simulink model "ex5"  (R2015a)
settings: Solver=ode45  StartTime=0.0  StopTime=100  RelTol=1e-3
values from neighbouring files (symbols this model uses):
  Kx = Kmpc(1,[1 2])    [ex5.m]
  Ky = Kmpc(1,3)    [ex5.m]
  r = 1    [ex5.m]
undefined symbols (not defined in the file or in its folder): Ad, Bd, Cd
libraries: simulink x1
settings Model: Creator=Xrisostomos  LastModifiedBy=Xrisostomos

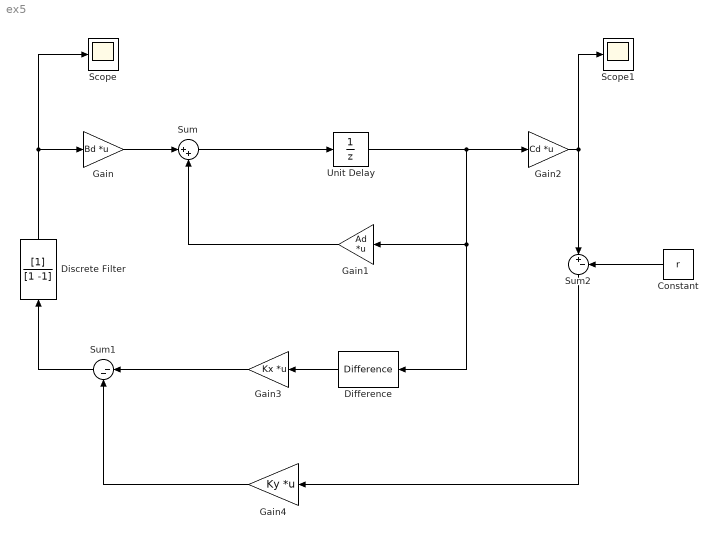
== system ex5 ==
  Constant : Constant  Value=r
  Difference : simulink/Discrete/Difference  ICPrevInput=0.0  InputProcessing=Inherited  OutMin=[]  OutMax=[]  OutDataType=fixdt(1, 16)  OutScaling=2^-10  DoSatur=off
  Discrete Filter : DiscreteFilter  Denominator=[1 -1]  SampleTime=2
  Gain : Gain  Gain=Bd  Multiplication=Matrix(K*u)
  Gain1 : Gain  Gain=Ad  Multiplication=Matrix(K*u)
  Gain2 : Gain  Gain=Cd  Multiplication=Matrix(K*u)
  Gain3 : Gain  Gain=Kx  Multiplication=Matrix(K*u)
  Gain4 : Gain  Gain=Ky  Multiplication=Matrix(K*u)
  Scope : Scope
  Scope1 : Scope
  Sum : Sum  Inputs=|++
  Sum1 : Sum  Inputs=|--
  Sum2 : Sum  Inputs=|+-
  Unit Delay : UnitDelay  SampleTime=-1
  wires:
  Gain1/1 -> Sum/2
  Sum/1 -> Unit Delay/1
  Unit Delay/1 -> Gain2/1, Difference/1, Gain1/1
  Difference/1 -> Gain3/1
  Gain3/1 -> Sum1/1
  Sum1/1 -> Discrete Filter/1
  Discrete Filter/1 -> Scope/1, Gain/1
  Gain/1 -> Sum/1
  Gain4/1 -> Sum1/2
  Constant/1 -> Sum2/2
  Gain2/1 -> Sum2/1, Scope1/1
  Sum2/1 -> Gain4/1
